simulink model "smomodel"  (Simulink 7.9)
settings: Solver=ode45  StartTime=0.0  StopTime=10.0  RelTol=1e-3
values from neighbouring files (symbols this model uses):
  A = zeros(5,5,K)    [aaushipcode.m]    (also in contsimu.m = [-betaX 0 0;      0 0 1;      0 0 -betaW]; disc2.m = [-betaX 0 0;      0 0 1;      0 0 -betaW]; discreteship.m = [-5.8/m 0 0;                0 0 1;                0 0 -2]; ncomputation.m = [K K;K*C1 K*C2])
  B = zeros(5,2,K)    [aaushipcode.m]    (also in contsimu.m = [1/m 0;      0 0;      0 1/I]; disc2.m = [1/m 0;      0 0;      0 1/I]; discreteship.m = [0.62/m 0.62/m;                0 0;                0.0305/I ; kalman.m = zeros(9,9,N))
  C = zeros(2,5,K)    [aaushipcode.m]    (also in contsimu.m = [1 0 0;      0 1 0]; disc2.m = [1 0 0;      0 1 0]; discreteship.m = [1 0 0;                0 1 0]; test2.m = [1 0 0;      0 1 0])
settings Model: Creator=Lunde  LastModifiedBy=Lunde

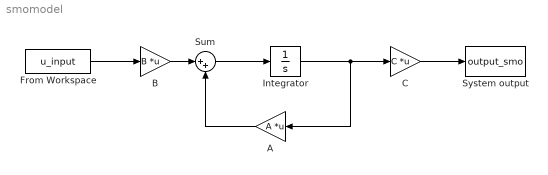
== system smomodel ==
  A : Gain  Gain=A  Multiplication=Matrix(K*u)
  B : Gain  Gain=B  Multiplication=Matrix(K*u)
  C : Gain  Gain=C  Multiplication=Matrix(K*u)
  From Workspace : FromWorkspace  VariableName=u_input  SampleTime=0
  Integrator : Integrator
  Sum : Sum  Inputs=|++
  System output : ToWorkspace  VariableName=output_smo  SampleTime=-1
  wires:
  Integrator/1 -> C/1, A/1
  A/1 -> Sum/2
  B/1 -> Sum/1
  Sum/1 -> Integrator/1
  C/1 -> System output/1
  From Workspace/1 -> B/1
